simulink model "Controllers_Simulation"  (R2023b)
settings: Solver=VariableStepAuto  StartTime=0.0  StopTime=10  RelTol=1e-3
settings Model: SimulationMode=accelerator  Creator=kagom  LastModifiedBy=xblcn
settings SolverCC: ZeroCrossAlgorithm=Adaptive  AlgebraicLoopSolver=LineSearch
settings OptimizationCC: EfficientMapNaN2IntZero=off
settings DebuggingCC: IgnoredZcDiagnostic=none  UnconnectedInputMsg=warning  UnconnectedOutputMsg=warning  UnconnectedLineMsg=warning
settings HardwareCC: TargetBitPerPointer=64  TargetBitPerSizeT=64  TargetBitPerPtrDiffT=64  TargetLongLongMode=on  TargetIntDivRoundTo=Zero  TargetEndianess=LittleEndian  TargetWordSize=64  TargetHWDeviceType=MATLAB Host  ProdEqTarget=off
settings ModelReferenceCC: EnableRefExpFcnMdlSchedulingChecks=on
settings SFSimCC: CustomCodeUndefinedFunction=UseInterfaceOnly
settings CodeAppCC: MaxIdLength=128
settings GRTTargetCC: TargetLangStandard=C89/C90 (ANSI)  CombineOutputUpdateFcns=off  GRTInterface=on

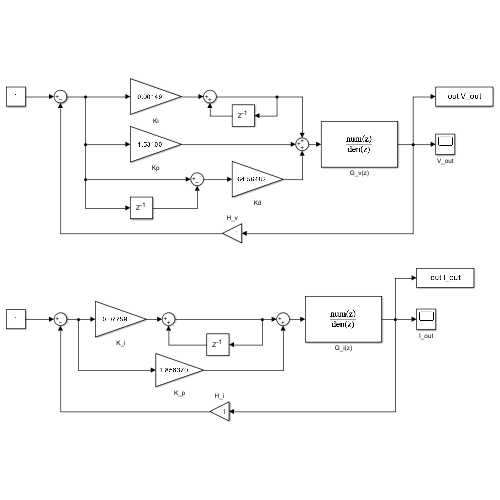
[thumbnail: Simulink's stored preview of the top-level diagram]
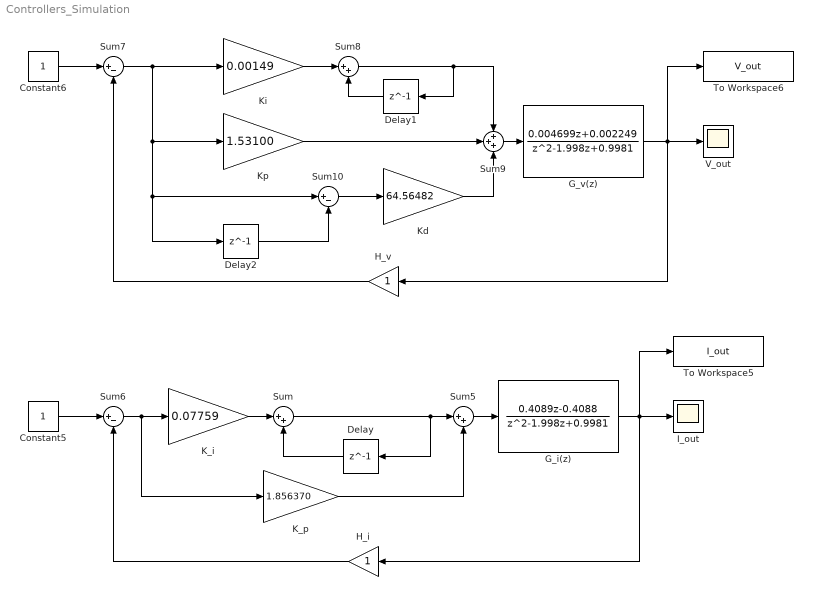
== system Controllers_Simulation ==
  Constant5 : Constant  VectorParams1D=off
  Constant6 : Constant  VectorParams1D=off
  Delay : Delay  DelayLength=1
  Delay1 : Delay  DelayLength=1
  Delay2 : Delay  DelayLength=1
  G_i(z) : DiscreteTransferFcn  Numerator=[0.4089 -0.4088]  Denominator=[1 -1.998 0.9981]
  G_v(z) : DiscreteTransferFcn  Numerator=[0.004699 0.002249]  Denominator=[1 -1.998 0.9981]
  H_i : Gain
  H_v : Gain
  I_out : Scope
  K_i : Gain  Gain=0.07759
  K_p : Gain  Gain=1.856370
  Kd : Gain  Gain=64.56482
  Ki : Gain  Gain=0.00149
  Kp : Gain  Gain=1.53100
  Sum : Sum  Inputs=|++
  Sum10 : Sum  Inputs=|+-
  Sum5 : Sum  Inputs=|++
  Sum6 : Sum  Inputs=|+-
  Sum7 : Sum  Inputs=|+-
  Sum8 : Sum  Inputs=|++
  Sum9 : Sum  Inputs=+++
  To Workspace5 : ToWorkspace  VariableName=I_out  SampleTime=8e-06
  To Workspace6 : ToWorkspace  VariableName=V_out  SampleTime=8e-06
  V_out : Scope
  wires:
  K_p/1 -> Sum5/2
  Sum6/1 -> K_i/1, K_p/1
  Delay/1 -> Sum/2
  K_i/1 -> Sum/1
  Sum/1 -> Sum5/1, Delay/1
  G_i(z)/1 -> To Workspace5/1, H_i/1, I_out/1
  H_i/1 -> Sum6/2
  Sum5/1 -> G_i(z)/1
  Constant5/1 -> Sum6/1
  G_v(z)/1 -> To Workspace6/1, V_out/1, H_v/1
  Constant6/1 -> Sum7/1
  H_v/1 -> Sum7/2
  Kp/1 -> Sum9/2
  Sum9/1 -> G_v(z)/1
  Delay2/1 -> Sum10/2
  Ki/1 -> Sum8/1
  Sum7/1 -> Delay2/1, Sum10/1, Kp/1, Ki/1
  Sum8/1 -> Delay1/1, Sum9/1
  Kd/1 -> Sum9/3
  Sum10/1 -> Kd/1
  Delay1/1 -> Sum8/2
